simulink model "Ex5"  (R2025b)
settings: Solver=VariableStepAuto  StartTime=0.0  StopTime=10.0  RelTol=1e-3

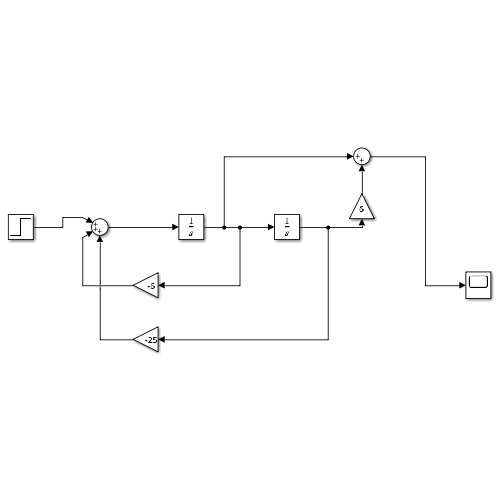
[thumbnail: Simulink's stored preview of the top-level diagram]
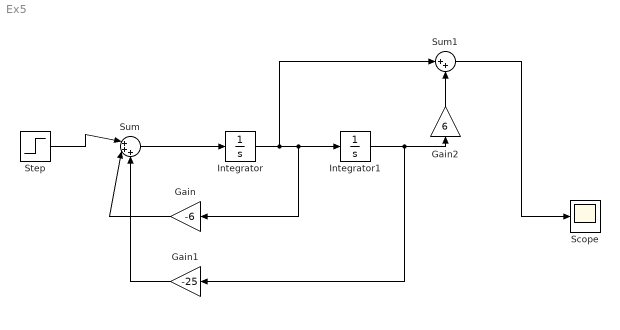
== system Ex5 ==
  Gain : Gain  Gain=-6
  Gain1 : Gain  Gain=-25
  Gain2 : Gain  Gain=6
  Integrator : Integrator
  Integrator1 : Integrator
  Scope : Scope
      settings: ActiveDisplayYMinimum=-0.087585981652732472  ActiveDisplayYMaximum=0.78827383487459235
  Step : Step  SampleTime=0
  Sum : Sum  Inputs=|+++
  Sum1 : Sum  Inputs=|++
  wires:
  Sum/1 -> Integrator/1
  Integrator/1 -> Sum1/1, Gain/1, Integrator1/1
  Gain/1 -> Sum/2
  Integrator1/1 -> Gain2/1, Gain1/1
  Gain1/1 -> Sum/3
  Step/1 -> Sum/1
  Gain2/1 -> Sum1/2
  Sum1/1 -> Scope/1
